simulink model "Optimization"  (R2021b)
settings: Solver=VariableStepAuto  StartTime=0.0  StopTime=10.0  RelTol=1e-3
model workspace (MAT data in the model file):
  Ixx = 1
  Iyy = Simulink.Parameter
  Iyy.DataType = 'auto'
  Iyy.Complexity = 'real'
  Iyy.Dimensions = [0 0]
  Izz = 1
libraries: slpidlib x4
settings Model: Creator=MahMooD  LastModifiedBy=MahMooD

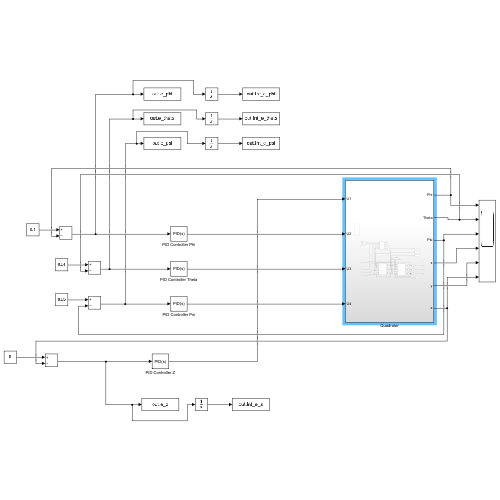
[thumbnail: Simulink's stored preview of the top-level diagram]
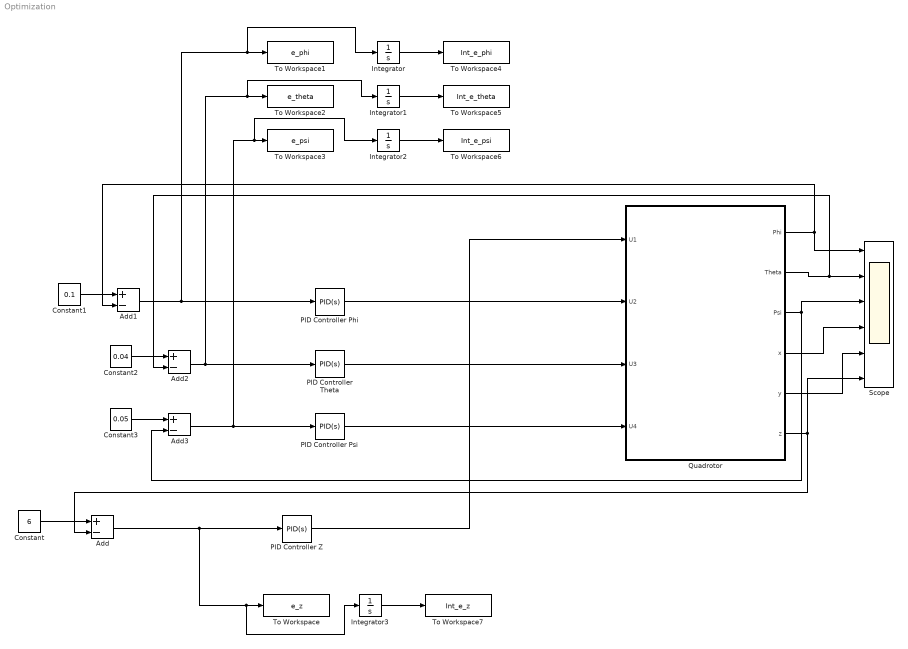
== system Optimization ==
  Add{,1..3} (4 alike) : Sum  Inputs=+-
  Constant : Constant  Value=6
  Constant1 : Constant  Value=0.1
  Constant2 : Constant  Value=0.04
  Constant3 : Constant  Value=0.05
  Integrator{,1..3} (4 alike) : Integrator
  PID Controller Phi : slpidlib/PID Controller  Controller=PID  Form=Parallel  TimeDomain=Continuous-time  UseExternalTs=off  SampleTime=-1  IntegratorMethod=Forward Euler  FilterMethod=Forward Euler  ControllerParametersSource=internal  P=0.0166019091775573  I=0.000617199200814389  D=0.0677385806674688  UseFilter=on  N=238.770606857548  TunerSelectOption=Transfer Function Based (PID Tuner App)  InitialConditionSource=internal  InitialConditionForIntegrator=0  InitialConditionForFilter=0  DifferentiatorICPrevScaledInput=0  ExternalReset=none  TrackingMode=off  Kt=1  LimitOutput=off  SatLimitsSource=internal  UpperSaturationLimit=inf  LowerSaturationLimit=-inf  LinearizeAsGain=on  AntiWindupMode=none  Kb=1  POutMin=[]  POutMax=[]  IOutMin=[]  IOutMax=[]  DOutMin=[]  DOutMax=[]  NOutMin=[]  NOutMax=[]  SumOutMin=[]  SumOutMax=[]  SaturationOutMin=[]  SaturationOutMax=[]  PParamMin=[]  PParamMax=[]  IParamMin=[]  IParamMax=[]  DParamMin=[]  DParamMax=[]  NParamMin=[]  NParamMax=[]  KbParamMin=[]  KbParamMax=[]  KtParamMin=[]  KtParamMax=[]  KbOutMin=[]  KbOutMax=[]  KtOutMin=[]  KtOutMax=[]  IntegratorOutMin=[]  IntegratorOutMax=[]  FilterOutMin=[]  FilterOutMax=[]  SumI1OutMin=[]  SumI1OutMax=[]  SumI2OutMin=[]  SumI2OutMax=[]  SumI3OutMin=[]  SumI3OutMax=[]  SumI4OutMin=[]  SumI4OutMax=[]  SumDOutMin=[]  SumDOutMax=[]  DifferentiatorOutMin=[]  DifferentiatorOutMax=[]  FilterDiffOutCoefMin=[]  FilterDiffOutCoefMax=[]  ReciprocalOutMin=[]  ReciprocalOutMax=[]  SumDenOutMin=[]  SumDenOutMax=[]  SumNumOutMin=[]  SumNumOutMax=[]  DivideOutMin=[]  DivideOutMax=[]  UdiffTsProdOutMin=[]  UdiffTsProdOutMax=[]  NTsProdOutMin=[]  NTsProdOutMax=[]  UintegralTsProdOutMin=[]  UintegralTsProdOutMax=[]  UngainTsProdOutMin=[]  UngainTsProdOutMax=[]  IntegratorContinuousStateAttributes=''  IntegratorStateMustResolveToSignalObject=off  IntegratorRTWStateStorageClass=Auto  FilterContinuousStateAttributes=''  FilterStateMustResolveToSignalObject=off  FilterRTWStateStorageClass=Auto  ParallelPVariant=InternalParameters  IdealPVariant=Disabled  IVariant=InternalParameters  DVariant=InternalParameters  IntegratorVariant=Continuous  SatVariant=Disabled  AWVariant=Passthrough  PCopyVariant=Disabled  TRVariant=Disabled  FdbkBlocksVariant=Forward  IdealPFdbkVariant=Disabled  SatFdbkVariant=Disabled  DerivativeFilterVariant=ContFilter  NVariant=InternalParameters  NCopyVariant=Disabled  FilterICVariant=InternalICsFilter  IntegratorICVariant=InternalICs  ExternalResetVariant=Disabled  TRSumVariant=Passthrough  SumFdbkVariant=Disabled  SumVariant=Sum_PID  TsampFilterVariant=InternalTs  TsampNgainVariant=Passthrough  TsampIntegralVariant=Passthrough  ExternalSaturationOutDataTypeStr=Inherit: Same as second input
  PID Controller Psi : slpidlib/PID Controller  Controller=PID  Form=Parallel  TimeDomain=Continuous-time  UseExternalTs=off  SampleTime=-1  IntegratorMethod=Forward Euler  FilterMethod=Forward Euler  ControllerParametersSource=internal  P=0.000884103470964375  I=6.9172864613183e-05  D=0.00267065329739963  UseFilter=on  N=21.9161221771913  TunerSelectOption=Transfer Function Based (PID Tuner App)  InitialConditionSource=internal  InitialConditionForIntegrator=0  InitialConditionForFilter=0  DifferentiatorICPrevScaledInput=0  ExternalReset=none  TrackingMode=off  Kt=1  LimitOutput=off  SatLimitsSource=internal  UpperSaturationLimit=inf  LowerSaturationLimit=-inf  LinearizeAsGain=on  AntiWindupMode=none  Kb=1  POutMin=[]  POutMax=[]  IOutMin=[]  IOutMax=[]  DOutMin=[]  DOutMax=[]  NOutMin=[]  NOutMax=[]  SumOutMin=[]  SumOutMax=[]  SaturationOutMin=[]  SaturationOutMax=[]  PParamMin=[]  PParamMax=[]  IParamMin=[]  IParamMax=[]  DParamMin=[]  DParamMax=[]  NParamMin=[]  NParamMax=[]  KbParamMin=[]  KbParamMax=[]  KtParamMin=[]  KtParamMax=[]  KbOutMin=[]  KbOutMax=[]  KtOutMin=[]  KtOutMax=[]  IntegratorOutMin=[]  IntegratorOutMax=[]  FilterOutMin=[]  FilterOutMax=[]  SumI1OutMin=[]  SumI1OutMax=[]  SumI2OutMin=[]  SumI2OutMax=[]  SumI3OutMin=[]  SumI3OutMax=[]  SumI4OutMin=[]  SumI4OutMax=[]  SumDOutMin=[]  SumDOutMax=[]  DifferentiatorOutMin=[]  DifferentiatorOutMax=[]  FilterDiffOutCoefMin=[]  FilterDiffOutCoefMax=[]  ReciprocalOutMin=[]  ReciprocalOutMax=[]  SumDenOutMin=[]  SumDenOutMax=[]  SumNumOutMin=[]  SumNumOutMax=[]  DivideOutMin=[]  DivideOutMax=[]  UdiffTsProdOutMin=[]  UdiffTsProdOutMax=[]  NTsProdOutMin=[]  NTsProdOutMax=[]  UintegralTsProdOutMin=[]  UintegralTsProdOutMax=[]  UngainTsProdOutMin=[]  UngainTsProdOutMax=[]  IntegratorContinuousStateAttributes=''  IntegratorStateMustResolveToSignalObject=off  IntegratorRTWStateStorageClass=Auto  FilterContinuousStateAttributes=''  FilterStateMustResolveToSignalObject=off  FilterRTWStateStorageClass=Auto  ParallelPVariant=InternalParameters  IdealPVariant=Disabled  IVariant=InternalParameters  DVariant=InternalParameters  IntegratorVariant=Continuous  SatVariant=Disabled  AWVariant=Passthrough  PCopyVariant=Disabled  TRVariant=Disabled  FdbkBlocksVariant=Forward  IdealPFdbkVariant=Disabled  SatFdbkVariant=Disabled  DerivativeFilterVariant=ContFilter  NVariant=InternalParameters  NCopyVariant=Disabled  FilterICVariant=InternalICsFilter  IntegratorICVariant=InternalICs  ExternalResetVariant=Disabled  TRSumVariant=Passthrough  SumFdbkVariant=Disabled  SumVariant=Sum_PID  TsampFilterVariant=InternalTs  TsampNgainVariant=Passthrough  TsampIntegralVariant=Passthrough  ExternalSaturationOutDataTypeStr=Inherit: Same as second input
  PID Controller Theta : slpidlib/PID Controller  Controller=PID  Form=Parallel  TimeDomain=Continuous-time  UseExternalTs=off  SampleTime=-1  IntegratorMethod=Forward Euler  FilterMethod=Forward Euler  ControllerParametersSource=internal  P=0.0298344301691438  I=0.00211790443594174  D=0.0852261154988147  UseFilter=on  N=300.594384562481  TunerSelectOption=Transfer Function Based (PID Tuner App)  InitialConditionSource=internal  InitialConditionForIntegrator=0  InitialConditionForFilter=0  DifferentiatorICPrevScaledInput=0  ExternalReset=none  TrackingMode=off  Kt=1  LimitOutput=off  SatLimitsSource=internal  UpperSaturationLimit=inf  LowerSaturationLimit=-inf  LinearizeAsGain=on  AntiWindupMode=none  Kb=1  POutMin=[]  POutMax=[]  IOutMin=[]  IOutMax=[]  DOutMin=[]  DOutMax=[]  NOutMin=[]  NOutMax=[]  SumOutMin=[]  SumOutMax=[]  SaturationOutMin=[]  SaturationOutMax=[]  PParamMin=[]  PParamMax=[]  IParamMin=[]  IParamMax=[]  DParamMin=[]  DParamMax=[]  NParamMin=[]  NParamMax=[]  KbParamMin=[]  KbParamMax=[]  KtParamMin=[]  KtParamMax=[]  KbOutMin=[]  KbOutMax=[]  KtOutMin=[]  KtOutMax=[]  IntegratorOutMin=[]  IntegratorOutMax=[]  FilterOutMin=[]  FilterOutMax=[]  SumI1OutMin=[]  SumI1OutMax=[]  SumI2OutMin=[]  SumI2OutMax=[]  SumI3OutMin=[]  SumI3OutMax=[]  SumI4OutMin=[]  SumI4OutMax=[]  SumDOutMin=[]  SumDOutMax=[]  DifferentiatorOutMin=[]  DifferentiatorOutMax=[]  FilterDiffOutCoefMin=[]  FilterDiffOutCoefMax=[]  ReciprocalOutMin=[]  ReciprocalOutMax=[]  SumDenOutMin=[]  SumDenOutMax=[]  SumNumOutMin=[]  SumNumOutMax=[]  DivideOutMin=[]  DivideOutMax=[]  UdiffTsProdOutMin=[]  UdiffTsProdOutMax=[]  NTsProdOutMin=[]  NTsProdOutMax=[]  UintegralTsProdOutMin=[]  UintegralTsProdOutMax=[]  UngainTsProdOutMin=[]  UngainTsProdOutMax=[]  IntegratorContinuousStateAttributes=''  IntegratorStateMustResolveToSignalObject=off  IntegratorRTWStateStorageClass=Auto  FilterContinuousStateAttributes=''  FilterStateMustResolveToSignalObject=off  FilterRTWStateStorageClass=Auto  ParallelPVariant=InternalParameters  IdealPVariant=Disabled  IVariant=InternalParameters  DVariant=InternalParameters  IntegratorVariant=Continuous  SatVariant=Disabled  AWVariant=Passthrough  PCopyVariant=Disabled  TRVariant=Disabled  FdbkBlocksVariant=Forward  IdealPFdbkVariant=Disabled  SatFdbkVariant=Disabled  DerivativeFilterVariant=ContFilter  NVariant=InternalParameters  NCopyVariant=Disabled  FilterICVariant=InternalICsFilter  IntegratorICVariant=InternalICs  ExternalResetVariant=Disabled  TRSumVariant=Passthrough  SumFdbkVariant=Disabled  SumVariant=Sum_PID  TsampFilterVariant=InternalTs  TsampNgainVariant=Passthrough  TsampIntegralVariant=Passthrough  ExternalSaturationOutDataTypeStr=Inherit: Same as second input
  PID Controller Z : slpidlib/PID Controller  Controller=PID  Form=Parallel  TimeDomain=Continuous-time  UseExternalTs=off  SampleTime=-1  IntegratorMethod=Forward Euler  FilterMethod=Forward Euler  ControllerParametersSource=internal  P=1  I=1  D=0  UseFilter=on  N=100  TunerSelectOption=Transfer Function Based (PID Tuner App)  InitialConditionSource=internal  InitialConditionForIntegrator=0  InitialConditionForFilter=0  DifferentiatorICPrevScaledInput=0  ExternalReset=none  TrackingMode=off  Kt=1  LimitOutput=off  SatLimitsSource=internal  UpperSaturationLimit=inf  LowerSaturationLimit=-inf  LinearizeAsGain=on  AntiWindupMode=none  Kb=1  POutMin=[]  POutMax=[]  IOutMin=[]  IOutMax=[]  DOutMin=[]  DOutMax=[]  NOutMin=[]  NOutMax=[]  SumOutMin=[]  SumOutMax=[]  SaturationOutMin=[]  SaturationOutMax=[]  PParamMin=[]  PParamMax=[]  IParamMin=[]  IParamMax=[]  DParamMin=[]  DParamMax=[]  NParamMin=[]  NParamMax=[]  KbParamMin=[]  KbParamMax=[]  KtParamMin=[]  KtParamMax=[]  KbOutMin=[]  KbOutMax=[]  KtOutMin=[]  KtOutMax=[]  IntegratorOutMin=[]  IntegratorOutMax=[]  FilterOutMin=[]  FilterOutMax=[]  SumI1OutMin=[]  SumI1OutMax=[]  SumI2OutMin=[]  SumI2OutMax=[]  SumI3OutMin=[]  SumI3OutMax=[]  SumI4OutMin=[]  SumI4OutMax=[]  SumDOutMin=[]  SumDOutMax=[]  DifferentiatorOutMin=[]  DifferentiatorOutMax=[]  FilterDiffOutCoefMin=[]  FilterDiffOutCoefMax=[]  ReciprocalOutMin=[]  ReciprocalOutMax=[]  SumDenOutMin=[]  SumDenOutMax=[]  SumNumOutMin=[]  SumNumOutMax=[]  DivideOutMin=[]  DivideOutMax=[]  UdiffTsProdOutMin=[]  UdiffTsProdOutMax=[]  NTsProdOutMin=[]  NTsProdOutMax=[]  UintegralTsProdOutMin=[]  UintegralTsProdOutMax=[]  UngainTsProdOutMin=[]  UngainTsProdOutMax=[]  IntegratorContinuousStateAttributes=''  IntegratorStateMustResolveToSignalObject=off  IntegratorRTWStateStorageClass=Auto  FilterContinuousStateAttributes=''  FilterStateMustResolveToSignalObject=off  FilterRTWStateStorageClass=Auto  ParallelPVariant=InternalParameters  IdealPVariant=Disabled  IVariant=InternalParameters  DVariant=InternalParameters  IntegratorVariant=Continuous  SatVariant=Disabled  AWVariant=Passthrough  PCopyVariant=Disabled  TRVariant=Disabled  FdbkBlocksVariant=Forward  IdealPFdbkVariant=Disabled  SatFdbkVariant=Disabled  DerivativeFilterVariant=ContFilter  NVariant=InternalParameters  NCopyVariant=Disabled  FilterICVariant=InternalICsFilter  IntegratorICVariant=InternalICs  ExternalResetVariant=Disabled  TRSumVariant=Passthrough  SumFdbkVariant=Disabled  SumVariant=Sum_PID  TsampFilterVariant=InternalTs  TsampNgainVariant=Passthrough  TsampIntegralVariant=Passthrough  ExternalSaturationOutDataTypeStr=Inherit: Same as second input
  Quadrotor : Subsystem
  Scope : Scope  NumInputPorts=6
  To Workspace : ToWorkspace  VariableName=e_z  SaveFormat=Timeseries  SampleTime=-1
  To Workspace1 : ToWorkspace  VariableName=e_phi  SaveFormat=Timeseries  SampleTime=-1
  To Workspace2 : ToWorkspace  VariableName=e_theta  SaveFormat=Timeseries  SampleTime=-1
  To Workspace3 : ToWorkspace  VariableName=e_psi  SaveFormat=Timeseries  SampleTime=-1
  To Workspace4 : ToWorkspace  VariableName=Int_e_phi  SaveFormat=Timeseries  SampleTime=-1
  To Workspace5 : ToWorkspace  VariableName=Int_e_theta  SaveFormat=Timeseries  SampleTime=-1
  To Workspace6 : ToWorkspace  VariableName=Int_e_psi  SaveFormat=Timeseries  SampleTime=-1
  To Workspace7 : ToWorkspace  VariableName=Int_e_z  SaveFormat=Timeseries  SampleTime=-1
  wires:
  PID Controller Z/1 -> Quadrotor/1(U1)
  PID Controller Theta/1 -> Quadrotor/3(U3)
  PID Controller Phi/1 -> Quadrotor/2(U2)
  PID Controller Psi/1 -> Quadrotor/4(U4)
  Quadrotor/2(Theta) -> Add2/2, Scope/2
  Add/1 -> Integrator3/1, To Workspace/1, PID Controller Z/1
  Constant/1 -> Add/1
  Quadrotor/1(Phi) -> Add1/2, Scope/1
  Quadrotor/3(Psi) -> Add3/2, Scope/3
  Quadrotor/4(x) -> Scope/4
  Quadrotor/5(y) -> Scope/5
  Quadrotor/6(z) -> Add/2, Scope/6
  Constant1/1 -> Add1/1
  Constant2/1 -> Add2/1
  Constant3/1 -> Add3/1
  Add2/1 -> Integrator1/1, To Workspace2/1, PID Controller Theta/1
  Add3/1 -> Integrator2/1, To Workspace3/1, PID Controller Psi/1
  Add1/1 -> Integrator/1, To Workspace1/1, PID Controller Phi/1
  Integrator/1 -> To Workspace4/1
  Integrator1/1 -> To Workspace5/1
  Integrator2/1 -> To Workspace6/1
  Integrator3/1 -> To Workspace7/1

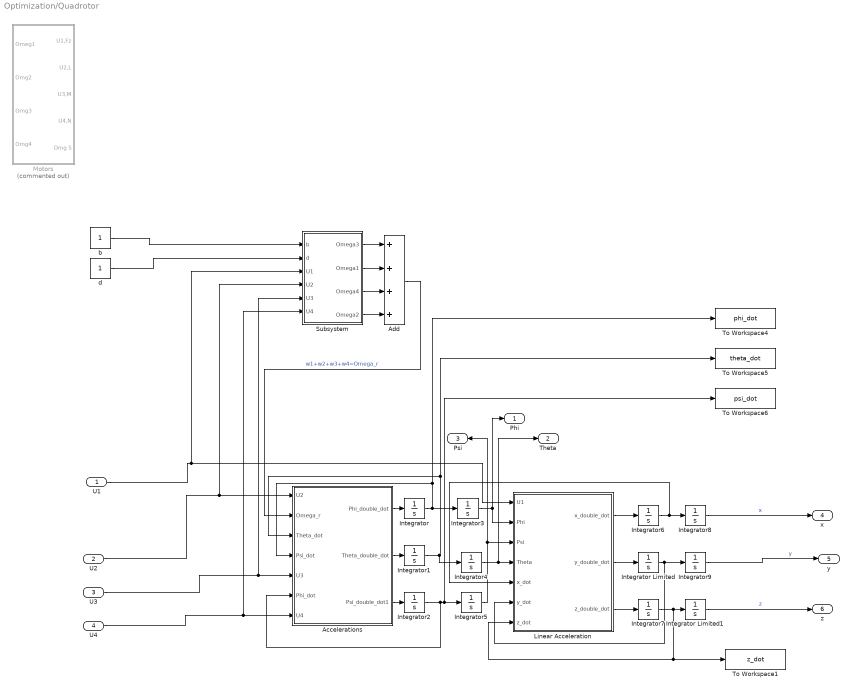
== system Optimization/Quadrotor ==
  U1 : Inport
  U2 : Inport  Port=2
  U3 : Inport  Port=3
  U4 : Inport  Port=4
  Accelerations : Subsystem
  Add : Sum  Inputs=++++
  Integrator{,1..9} (10 alike) : Integrator
  Integrator Limited : Integrator  LimitOutput=on  UpperSaturationLimit=1  LowerSaturationLimit=0
  Integrator Limited1 : Integrator  LimitOutput=on  UpperSaturationLimit=1  LowerSaturationLimit=0
  Linear Acceleration : Subsystem
  Motors : Subsystem  Commented=on
  Subsystem : Subsystem
  To Workspace1 : ToWorkspace  VariableName=z_dot  SaveFormat=Timeseries  SampleTime=-1
  To Workspace4 : ToWorkspace  VariableName=phi_dot  SaveFormat=Timeseries  SampleTime=-1
  To Workspace5 : ToWorkspace  VariableName=theta_dot  SaveFormat=Timeseries  SampleTime=-1
  To Workspace6 : ToWorkspace  VariableName=psi_dot  SaveFormat=Timeseries  SampleTime=-1
  b : Constant
  d : Constant
  Phi : Outport
  Theta : Outport  Port=2
  Psi : Outport  Port=3
  x : Outport  Port=4
  y : Outport  Port=5
  z : Outport  Port=6
  wires:
  Accelerations/1(Phi_double_dot) -> Integrator/1
  Integrator2/1 -> To Workspace6/1, Integrator5/1, Accelerations/6(Phi_dot)
  Accelerations/2(Theta_double_dot) -> Integrator1/1
  Integrator/1 -> Integrator3/1, To Workspace4/1, Accelerations/4(Psi_dot)
  Integrator Limited1/1 -> z/1  "z"
  Accelerations/3(Psi_double_dot1) -> Integrator2/1
  Integrator1/1 -> Integrator4/1, To Workspace5/1, Accelerations/3(Theta_dot)
  Integrator6/1 -> Linear Acceleration/5(x_dot), Integrator8/1
  Integrator Limited/1 -> Integrator9/1, Linear Acceleration/6(y_dot)
  Linear Acceleration/2(y_double_dot) -> Integrator Limited/1
  Integrator5/1 -> Psi/1, Linear Acceleration/3(Psi)
  Integrator7/1 -> To Workspace1/1, Linear Acceleration/7(z_dot), Integrator Limited1/1
  Integrator4/1 -> Theta/1, Linear Acceleration/4(Theta)
  Integrator3/1 -> Phi/1, Linear Acceleration/2(Phi)
  Linear Acceleration/1(x_double_dot) -> Integrator6/1
  Linear Acceleration/3(z_double_dot) -> Integrator7/1
  Integrator8/1 -> x/1  "x"
  Integrator9/1 -> y/1  "y"
  U4/1 -> Accelerations/7(U4), Subsystem/6(U4)
  U3/1 -> Accelerations/5(U3), Subsystem/5(U3)
  U2/1 -> Accelerations/1(U2), Subsystem/4(U2)
  U1/1 -> Linear Acceleration/1(U1), Subsystem/3(U1)
  b/1 -> Subsystem/1(b)
  d/1 -> Subsystem/2(d)
  Subsystem/1(Omega3) -> Add/1
  Subsystem/2(Omega1) -> Add/2
  Subsystem/3(Omega4) -> Add/3
  Subsystem/4(Omega2) -> Add/4
  Add/1 -> Accelerations/2(Omega_r)  "w1+w2+w3+w4=Omega_r"

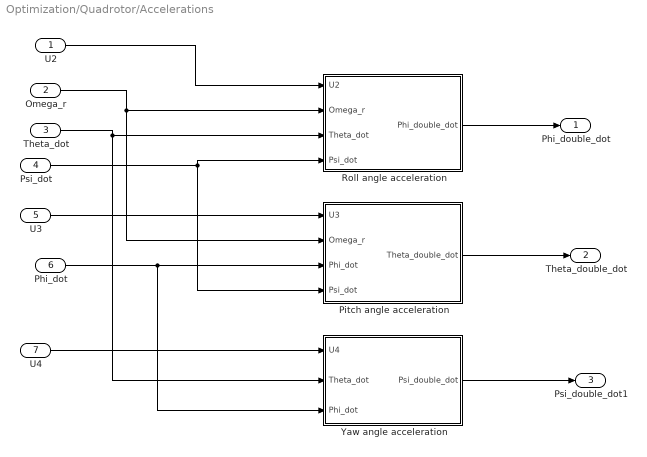
== system Optimization/Quadrotor/Accelerations ==
  U2 : Inport
  Omega_r : Inport  Port=2
  Theta_dot : Inport  Port=3
  Psi_dot : Inport  Port=4
  U3 : Inport  Port=5
  Phi_dot : Inport  Port=6
  U4 : Inport  Port=7
  Pitch angle acceleration : Subsystem
  Roll angle acceleration : Subsystem
  Yaw angle acceleration : Subsystem
  Phi_double_dot : Outport
  Theta_double_dot : Outport  Port=2
  Psi_double_dot1 : Outport  Port=3
  wires:
  Roll angle acceleration/1(Phi_double_dot) -> Phi_double_dot/1
  Theta_dot/1 -> Roll angle acceleration/3(Theta_dot), Yaw angle acceleration/2(Theta_dot)
  Omega_r/1 -> Pitch angle acceleration/2(Omega_r), Roll angle acceleration/2(Omega_r)
  Psi_dot/1 -> Pitch angle acceleration/4(Psi_dot), Roll angle acceleration/4(Psi_dot)
  Phi_dot/1 -> Yaw angle acceleration/3(Phi_dot), Pitch angle acceleration/3(Phi_dot)
  U3/1 -> Pitch angle acceleration/1(U3)
  Pitch angle acceleration/1(Theta_double_dot) -> Theta_double_dot/1
  Yaw angle acceleration/1(Psi_double_dot) -> Psi_double_dot1/1
  U4/1 -> Yaw angle acceleration/1(U4)
  U2/1 -> Roll angle acceleration/1(U2)

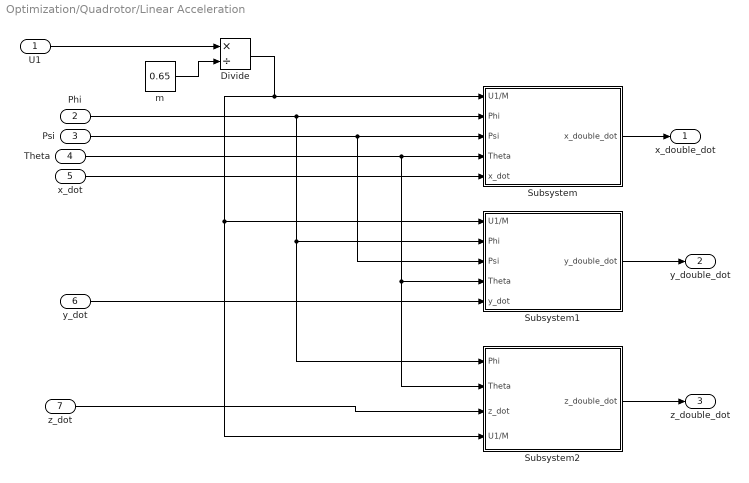
== system Optimization/Quadrotor/Linear Acceleration ==
  U1 : Inport
  Phi : Inport  Port=2
  Psi : Inport  Port=3
  Theta : Inport  Port=4
  x_dot : Inport  Port=5
  y_dot : Inport  Port=6
  z_dot : Inport  Port=7
  Divide : Product  Inputs=*/
  Subsystem : Subsystem
  Subsystem1 : Subsystem
  Subsystem2 : Subsystem
  m : Constant  Value=0.65
  x_double_dot : Outport
  y_double_dot : Outport  Port=2
  z_double_dot : Outport  Port=3
  wires:
  Phi/1 -> Subsystem2/1(Phi), Subsystem1/2(Phi), Subsystem/2(Phi)
  m/1 -> Divide/2
  Divide/1 -> Subsystem/1(U1/M), Subsystem2/4(U1/M), Subsystem1/1(U1/M)
  y_dot/1 -> Subsystem1/5(y_dot)
  Theta/1 -> Subsystem1/4(Theta), Subsystem2/2(Theta), Subsystem/4(Theta)
  Psi/1 -> Subsystem1/3(Psi), Subsystem/3(Psi)
  Subsystem1/1(y_double_dot) -> y_double_dot/1
  x_dot/1 -> Subsystem/5(x_dot)
  z_dot/1 -> Subsystem2/3(z_dot)
  Subsystem2/1(z_double_dot) -> z_double_dot/1
  Subsystem/1(x_double_dot) -> x_double_dot/1
  U1/1 -> Divide/1

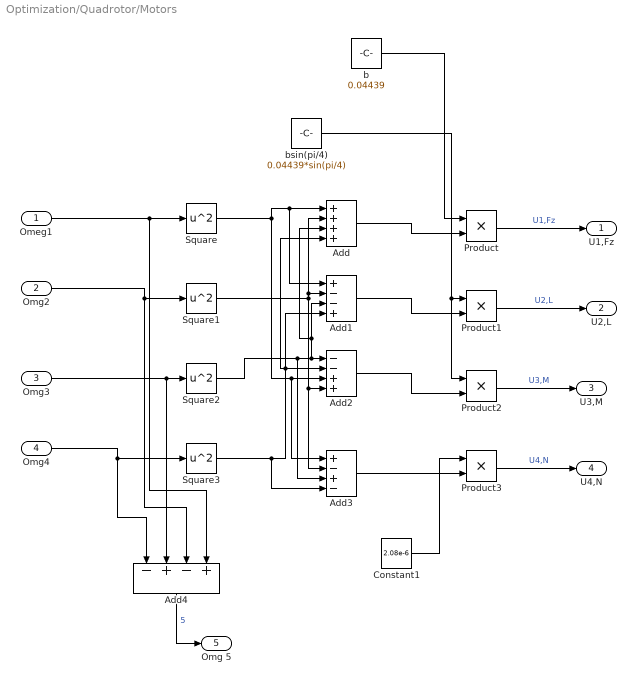
== system Optimization/Quadrotor/Motors ==
  Omeg1 : Inport
  Omg2 : Inport  Port=2
  Omg3 : Inport  Port=3
  Omg4 : Inport  Port=4
  Add : Sum  Inputs=++++
  Add1 : Sum  Inputs=+--+
  Add2 : Sum  Inputs=--++
  Add3 : Sum  Inputs=+-+-
  Add4 : Sum  Inputs=-+-+
  Constant1 : Constant  Value=2.08e-6
  Product{,1..3} (4 alike) : Product
  Square{,1..3} (4 alike) : Math  Operator=square  SaturateOnIntegerOverflow=on
  b : Constant  Value=0.04439
  bsin(pi/4) : Constant  Value=0.04439*sin(pi/4)
  U1,Fz : Outport
  U2,L : Outport  Port=2
  U3,M : Outport  Port=3
  U4,N : Outport  Port=4
  Omg 5 : Outport  Port=5
  wires:
  Constant1/1 -> Product3/1
  Add2/1 -> Product2/2
  Add/1 -> Product/2
  Add1/1 -> Product1/2
  Omg4/1 -> Add4/1, Square3/1
  Square2/1 -> Add1/3, Add/3, Add2/1, Add3/3
  Omg3/1 -> Add4/2, Square2/1
  Add3/1 -> Product3/2
  Square3/1 -> Add2/2, Add1/4, Add/4, Add3/4
  Product/1 -> U1,Fz/1  "U1,Fz"
  Add4/1 -> Omg 5/1  "5"
  Omg2/1 -> Add4/3, Square1/1
  Product3/1 -> U4,N/1  "U4,N"
  b/1 -> Product/1
  Product2/1 -> U3,M/1  "U3,M"
  bsin(pi/4)/1 -> Product2/1, Product1/1
  Product1/1 -> U2,L/1  "U2,L"
  Omeg1/1 -> Add4/4, Square/1
  Square1/1 -> Add3/2, Add2/4, Add/2, Add1/2
  Square/1 -> Add2/3, Add3/1, Add1/1, Add/1

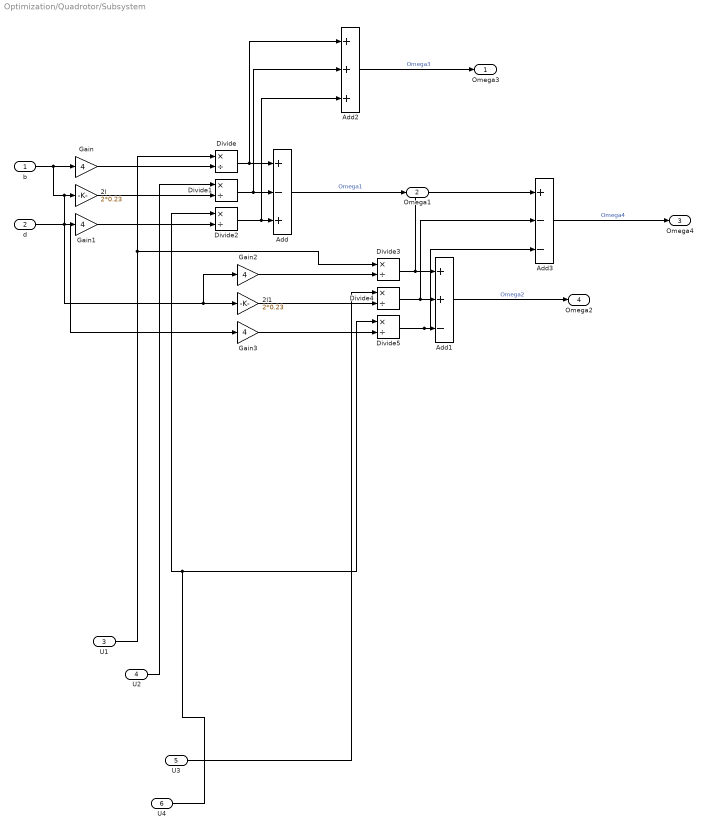
== system Optimization/Quadrotor/Subsystem ==
  b : Inport
  d : Inport  Port=2
  U1 : Inport  Port=3
  U2 : Inport  Port=4
  U3 : Inport  Port=5
  U4 : Inport  Port=6
  2l : Gain  Gain=2*0.23
  2l1 : Gain  Gain=2*0.23
  Add : Sum  Inputs=+-+
  Add1 : Sum  Inputs=++-
  Add2 : Sum  Inputs=+++
  Add3 : Sum  Inputs=+--
  Divide{,1..5} (6 alike) : Product  Inputs=*/
  Gain{,1..3} (4 alike) : Gain  Gain=4
  Omega3 : Outport
  Omega1 : Outport  Port=2
  Omega4 : Outport  Port=3
  Omega2 : Outport  Port=4
  wires:
  Divide1/1 -> Add/2, Add2/2
  b/1 -> Gain2/1, 2l1/1, 2l/1, Gain/1
  Divide/1 -> Add/1, Add2/1
  Divide5/1 -> Add3/3, Add1/3
  Gain/1 -> Divide/2
  Divide4/1 -> Add1/2, Add3/2
  Divide2/1 -> Add2/3, Add/3
  U2/1 -> Divide1/1
  d/1 -> Gain3/1, Gain1/1
  Gain3/1 -> Divide5/2
  Divide3/1 -> Add3/1, Add1/1
  2l/1 -> Divide1/2
  Gain1/1 -> Divide2/2
  Gain2/1 -> Divide3/2
  Add/1 -> Omega1/1  "Omega1"
  2l1/1 -> Divide4/2
  Add2/1 -> Omega3/1  "Omega3"
  U4/1 -> Divide5/1, Divide2/1
  U3/1 -> Divide4/1
  Add3/1 -> Omega4/1  "Omega4"
  U1/1 -> Divide3/1, Divide/1
  Add1/1 -> Omega2/1  "Omega2"

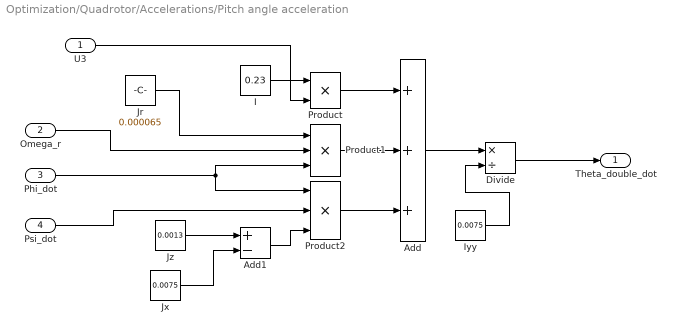
== system Optimization/Quadrotor/Accelerations/Pitch angle acceleration ==
  U3 : Inport
  Omega_r : Inport  Port=2
  Phi_dot : Inport  Port=3
  Psi_dot : Inport  Port=4
  Add : Sum  Inputs=+++
  Add1 : Sum  Inputs=+-
  Divide : Product  Inputs=*/
  I : Constant  Value=0.23
  Iyy : Constant  Value=0.0075
  Jr : Constant  Value=0.000065
  Jx : Constant  Value=0.0075
  Jz : Constant  Value=0.0013
  Product : Product
  Product1 : Product  Inputs=3
  Product2 : Product  Inputs=3
  Theta_double_dot : Outport
  wires:
  Omega_r/1 -> Product1/2
  U3/1 -> Product/2
  Phi_dot/1 -> Product1/3, Product2/1
  Divide/1 -> Theta_double_dot/1
  Jr/1 -> Product1/1
  Add/1 -> Divide/1
  Product1/1 -> Add/2
  Iyy/1 -> Divide/2
  Psi_dot/1 -> Product2/2
  Product2/1 -> Add/3
  I/1 -> Product/1
  Add1/1 -> Product2/3
  Product/1 -> Add/1
  Jz/1 -> Add1/1
  Jx/1 -> Add1/2

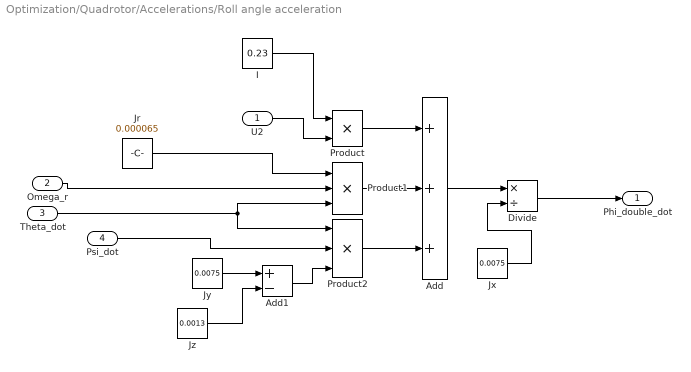
== system Optimization/Quadrotor/Accelerations/Roll angle acceleration ==
  U2 : Inport
  Omega_r : Inport  Port=2
  Theta_dot : Inport  Port=3
  Psi_dot : Inport  Port=4
  Add : Sum  Inputs=+++
  Add1 : Sum  Inputs=+-
  Divide : Product  Inputs=*/
  I : Constant  Value=0.23
  Jr : Constant  Value=0.000065
  Jx : Constant  Value=0.0075
  Jy : Constant  Value=0.0075
  Jz : Constant  Value=0.0013
  Product : Product
  Product1 : Product  Inputs=3
  Product2 : Product  Inputs=3
  Phi_double_dot : Outport
  wires:
  Jz/1 -> Add1/2
  Product/1 -> Add/1
  Jy/1 -> Add1/1
  Add1/1 -> Product2/3
  I/1 -> Product/1
  Product2/1 -> Add/3
  Psi_dot/1 -> Product2/2
  Jx/1 -> Divide/2
  Product1/1 -> Add/2
  Add/1 -> Divide/1
  Jr/1 -> Product1/1
  Divide/1 -> Phi_double_dot/1
  Theta_dot/1 -> Product1/3, Product2/1
  U2/1 -> Product/2
  Omega_r/1 -> Product1/2

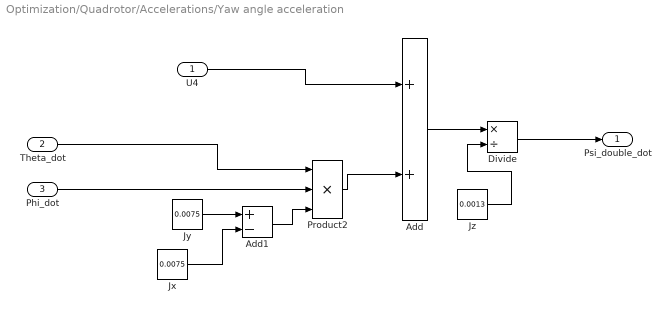
== system Optimization/Quadrotor/Accelerations/Yaw angle acceleration ==
  U4 : Inport
  Theta_dot : Inport  Port=2
  Phi_dot : Inport  Port=3
  Add : Sum
  Add1 : Sum  Inputs=+-
  Divide : Product  Inputs=*/
  Jx : Constant  Value=0.0075
  Jy : Constant  Value=0.0075
  Jz : Constant  Value=0.0013
  Product2 : Product  Inputs=3
  Psi_double_dot : Outport
  wires:
  Jx/1 -> Add1/2
  Jy/1 -> Add1/1
  Add1/1 -> Product2/3
  Product2/1 -> Add/2
  Phi_dot/1 -> Product2/2
  Jz/1 -> Divide/2
  Add/1 -> Divide/1
  Divide/1 -> Psi_double_dot/1
  Theta_dot/1 -> Product2/1
  U4/1 -> Add/1

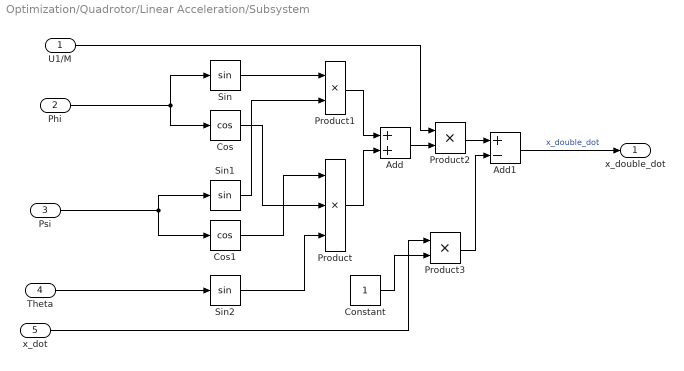
== system Optimization/Quadrotor/Linear Acceleration/Subsystem ==
  U1/M : Inport
  Phi : Inport  Port=2
  Psi : Inport  Port=3
  Theta : Inport  Port=4
  x_dot : Inport  Port=5
  Add : Sum
  Add1 : Sum  Inputs=+-
  Constant : Constant
  Cos : Trigonometry  Operator=cos
  Cos1 : Trigonometry  Operator=cos
  Product : Product  Inputs=3
  Product1 : Product
  Product2 : Product
  Product3 : Product
  Sin : Trigonometry
  Sin1 : Trigonometry
  Sin2 : Trigonometry
  x_double_dot : Outport
  wires:
  Product2/1 -> Add1/1
  Product/1 -> Add/2
  Phi/1 -> Sin/1, Cos/1
  Sin/1 -> Product1/1
  Constant/1 -> Product3/2
  x_dot/1 -> Product3/1
  Cos1/1 -> Product/1
  Sin2/1 -> Product/3
  Sin1/1 -> Product1/2
  Product3/1 -> Add1/2
  Psi/1 -> Cos1/1, Sin1/1
  Cos/1 -> Product/2
  Product1/1 -> Add/1
  Add/1 -> Product2/2
  Add1/1 -> x_double_dot/1  "x_double_dot"
  Theta/1 -> Sin2/1
  U1/M/1 -> Product2/1

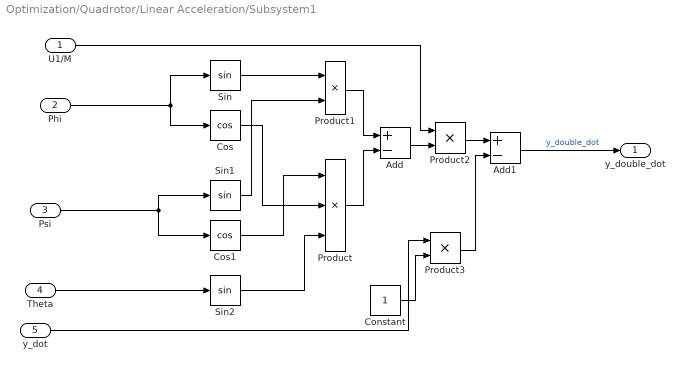
== system Optimization/Quadrotor/Linear Acceleration/Subsystem1 ==
  U1/M : Inport
  Phi : Inport  Port=2
  Psi : Inport  Port=3
  Theta : Inport  Port=4
  y_dot : Inport  Port=5
  Add : Sum  Inputs=+-
  Add1 : Sum  Inputs=+-
  Constant : Constant
  Cos : Trigonometry  Operator=cos
  Cos1 : Trigonometry  Operator=cos
  Product : Product  Inputs=3
  Product1 : Product
  Product2 : Product
  Product3 : Product
  Sin : Trigonometry
  Sin1 : Trigonometry
  Sin2 : Trigonometry
  y_double_dot : Outport
  wires:
  U1/M/1 -> Product2/1
  Theta/1 -> Sin2/1
  Add1/1 -> y_double_dot/1  "y_double_dot"
  Add/1 -> Product2/2
  Product1/1 -> Add/1
  Cos/1 -> Product/2
  Psi/1 -> Sin1/1, Cos1/1
  Product3/1 -> Add1/2
  Sin1/1 -> Product1/2
  Sin2/1 -> Product/3
  Cos1/1 -> Product/1
  y_dot/1 -> Product3/1
  Constant/1 -> Product3/2
  Sin/1 -> Product1/1
  Phi/1 -> Cos/1, Sin/1
  Product/1 -> Add/2
  Product2/1 -> Add1/1

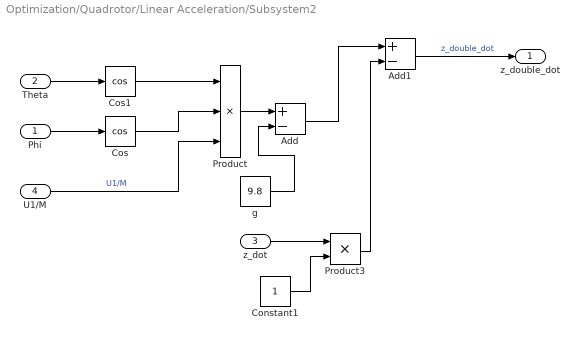
== system Optimization/Quadrotor/Linear Acceleration/Subsystem2 ==
  Phi : Inport
  Theta : Inport  Port=2
  z_dot : Inport  Port=3
  U1/M : Inport  Port=4
  Add : Sum  Inputs=+-
  Add1 : Sum  Inputs=+-
  Constant1 : Constant
  Cos : Trigonometry  Operator=cos
  Cos1 : Trigonometry  Operator=cos
  Product : Product  Inputs=3
  Product3 : Product
  g : Constant  Value=9.8
  z_double_dot : Outport
  wires:
  Add/1 -> Add1/1
  Phi/1 -> Cos/1
  Cos1/1 -> Product/1
  Product3/1 -> Add1/2
  Add1/1 -> z_double_dot/1  "z_double_dot"
  Theta/1 -> Cos1/1
  Product/1 -> Add/1
  g/1 -> Add/2
  z_dot/1 -> Product3/1
  Constant1/1 -> Product3/2
  U1/M/1 -> Product/3  "U1/M"
  Cos/1 -> Product/2
